simulink model "QuadCopter"  (R2024a)
settings: Solver=VariableStepAuto  StartTime=0.0  StopTime=Tsim  RelTol=1e-3
values from neighbouring files (symbols this model uses):
  l = size(Aa,2)    [RobustControl.m]
undefined symbols (not defined in the file or in its folder): b, d, g, Ixx, Iyy, Izz, Jr, m, x0
settings Model: Creator=giuco  LastModifiedBy=giuco

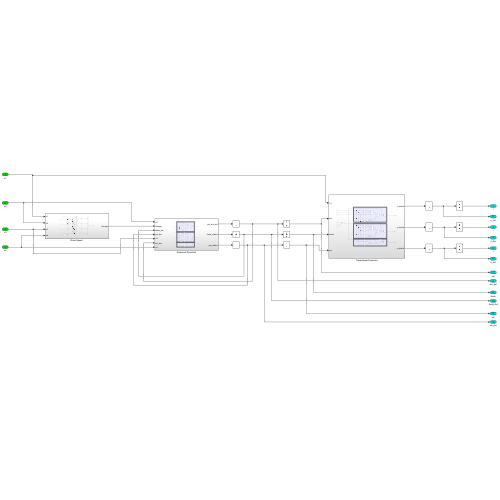
[thumbnail: Simulink's stored preview of the top-level diagram]
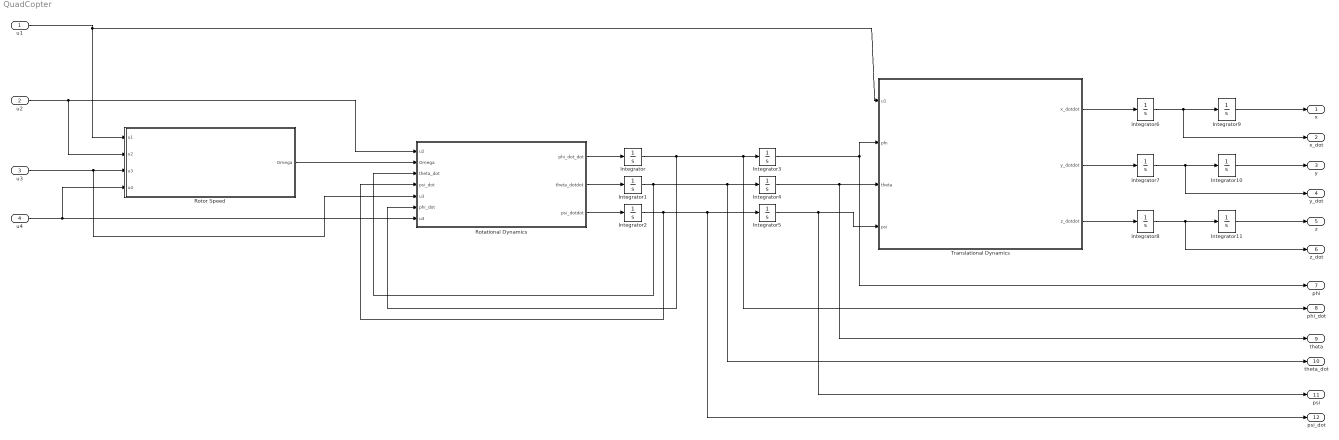
== system QuadCopter ==
  u1 : Inport
  u2 : Inport  Port=2
  u3 : Inport  Port=3
  u4 : Inport  Port=4
  Integrator : Integrator  InitialCondition=x0(2)
  Integrator1 : Integrator  InitialCondition=x0(4)
  Integrator10 : Integrator  InitialCondition=x0(9)
  Integrator11 : Integrator  InitialCondition=x0(11)
  Integrator2 : Integrator  InitialCondition=x0(6)
  Integrator3 : Integrator  InitialCondition=x0(1)
  Integrator4 : Integrator  InitialCondition=x0(3)
  Integrator5 : Integrator  InitialCondition=x0(5)
  Integrator6 : Integrator  InitialCondition=x0(8)
  Integrator7 : Integrator  InitialCondition=x0(10)
  Integrator8 : Integrator  InitialCondition=x0(12)
  Integrator9 : Integrator  InitialCondition=x0(7)
  Rotational Dynamics : Subsystem
  "Rotor Speed " : Subsystem
  Translational Dynamics : Subsystem
  x : Outport
  x_dot : Outport  Port=2
  y : Outport  Port=3
  y_dot : Outport  Port=4
  z : Outport  Port=5
  z_dot : Outport  Port=6
  phi : Outport  Port=7
  phi_dot : Outport  Port=8
  theta : Outport  Port=9
  theta_dot : Outport  Port=10
  psi : Outport  Port=11
  psi_dot : Outport  Port=12
  wires:
  u4/1 -> Rotational Dynamics/7(u4), "Rotor Speed "/4(u4)
  u2/1 -> Rotational Dynamics/1(u2), "Rotor Speed "/2(u2)
  Rotational Dynamics/1(phi_dot_dot) -> Integrator/1
  "Rotor Speed "/1(Omega) -> Rotational Dynamics/2(Omega)
  Integrator4/1 -> theta/1, Translational Dynamics/3(theta)
  Translational Dynamics/1(x_dotdot) -> Integrator6/1
  Rotational Dynamics/2(theta_dotdot) -> Integrator1/1
  Integrator5/1 -> psi/1, Translational Dynamics/4(psi)
  u1/1 -> "Rotor Speed "/1(u1), Translational Dynamics/1(u1)
  Integrator7/1 -> y_dot/1, Integrator10/1
  Integrator3/1 -> phi/1, Translational Dynamics/2(phi)
  Translational Dynamics/2(y_dotdot) -> Integrator7/1
  Integrator9/1 -> x/1
  Integrator1/1 -> theta_dot/1, Integrator4/1, Rotational Dynamics/3(theta_dot)
  Integrator10/1 -> y/1
  Integrator2/1 -> psi_dot/1, Integrator5/1, Rotational Dynamics/4(psi_dot)
  u3/1 -> "Rotor Speed "/3(u3), Rotational Dynamics/5(u3)
  Integrator6/1 -> x_dot/1, Integrator9/1
  Integrator/1 -> Rotational Dynamics/6(phi_dot), phi_dot/1, Integrator3/1
  Integrator8/1 -> z_dot/1, Integrator11/1
  Rotational Dynamics/3(psi_dotdot) -> Integrator2/1
  Translational Dynamics/3(z_dotdot) -> Integrator8/1
  Integrator11/1 -> z/1

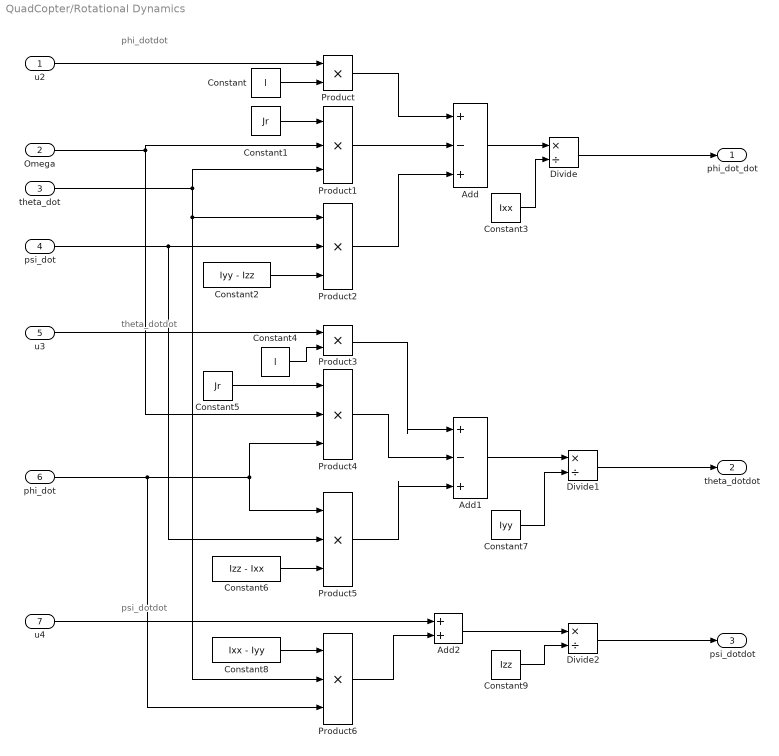
== system QuadCopter/Rotational Dynamics ==
  note: phi_dotdot
  note: theta_dotdot
  note: psi_dotdot
  u2 : Inport
  Omega : Inport  Port=2
  theta_dot : Inport  Port=3
  psi_dot : Inport  Port=4
  u3 : Inport  Port=5
  phi_dot : Inport  Port=6
  u4 : Inport  Port=7
  Add : Sum  Inputs=+-+
  Add1 : Sum  Inputs=+-+
  Add2 : Sum
  Constant : Constant  Value=l
  Constant1 : Constant  Value=Jr
  Constant2 : Constant  Value=Iyy - Izz
  Constant3 : Constant  Value=Ixx
  Constant4 : Constant  Value=l
  Constant5 : Constant  Value=Jr
  Constant6 : Constant  Value=Izz - Ixx
  Constant7 : Constant  Value=Iyy
  Constant8 : Constant  Value=Ixx - Iyy
  Constant9 : Constant  Value=Izz
  Divide : Product  Inputs=*/
  Divide1 : Product  Inputs=*/
  Divide2 : Product  Inputs=*/
  Product : Product
  Product{1..2,4..6} (5 alike) : Product  Inputs=3
  Product3 : Product
  phi_dot_dot : Outport
  theta_dotdot : Outport  Port=2
  psi_dotdot : Outport  Port=3
  wires:
  u2/1 -> Product/1
  Constant/1 -> Product/2
  Omega/1 -> Product1/2, Product4/2
  Constant1/1 -> Product1/1
  theta_dot/1 -> Product1/3, Product2/1, Product6/2
  psi_dot/1 -> Product5/2, Product2/2
  Constant2/1 -> Product2/3
  Product1/1 -> Add/2
  Product/1 -> Add/1
  Product2/1 -> Add/3
  Add/1 -> Divide/1
  Divide/1 -> phi_dot_dot/1
  Constant3/1 -> Divide/2
  u3/1 -> Product3/1
  Constant4/1 -> Product3/2
  Constant5/1 -> Product4/1
  phi_dot/1 -> Product4/3, Product5/1, Product6/3
  Constant6/1 -> Product5/3
  Product4/1 -> Add1/2
  Product3/1 -> Add1/1
  Product5/1 -> Add1/3
  Add1/1 -> Divide1/1
  Constant7/1 -> Divide1/2
  Divide1/1 -> theta_dotdot/1
  Constant8/1 -> Product6/1
  u4/1 -> Add2/1
  Product6/1 -> Add2/2
  Add2/1 -> Divide2/1
  Constant9/1 -> Divide2/2
  Divide2/1 -> psi_dotdot/1

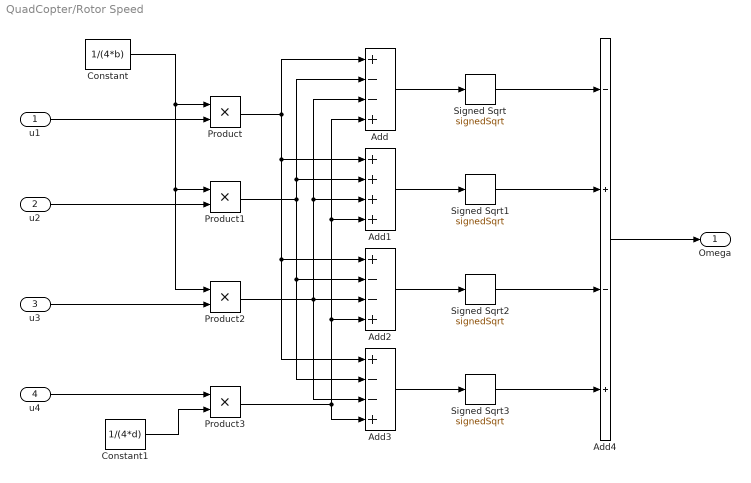
== system QuadCopter/Rotor Speed  ==
  u1 : Inport
  u2 : Inport  Port=2
  u3 : Inport  Port=3
  u4 : Inport  Port=4
  Add : Sum  Inputs=+--+
  Add1 : Sum  Inputs=++++
  Add2 : Sum  Inputs=+--+
  Add3 : Sum  Inputs=+--+
  Add4 : Sum  Inputs=-+-+
  Constant : Constant  Value=1/(4*b)
  Constant1 : Constant  Value=1/(4*d)
  Product{,1..3} (4 alike) : Product
  Signed Sqrt{,1..3} (4 alike) : Sqrt  Operator=signedSqrt
  Omega : Outport
  wires:
  u1/1 -> Product/2
  Constant/1 -> Product/1, Product1/1, Product2/1
  u2/1 -> Product1/2
  u3/1 -> Product2/2
  u4/1 -> Product3/1
  Constant1/1 -> Product3/2
  Product/1 -> Add3/1, Add2/1, Add1/1, Add/1
  Product1/1 -> Add2/2, Add3/2, Add1/2, Add/2
  Product2/1 -> Add2/3, Add1/3, Add/3, Add3/3
  Product3/1 -> Add3/4, Add2/4, Add/4, Add1/4
  Add/1 -> Signed Sqrt/1
  Add1/1 -> Signed Sqrt1/1
  Add2/1 -> Signed Sqrt2/1
  Add3/1 -> Signed Sqrt3/1
  Signed Sqrt/1 -> Add4/1
  Signed Sqrt1/1 -> Add4/2
  Signed Sqrt2/1 -> Add4/3
  Signed Sqrt3/1 -> Add4/4
  Add4/1 -> Omega/1

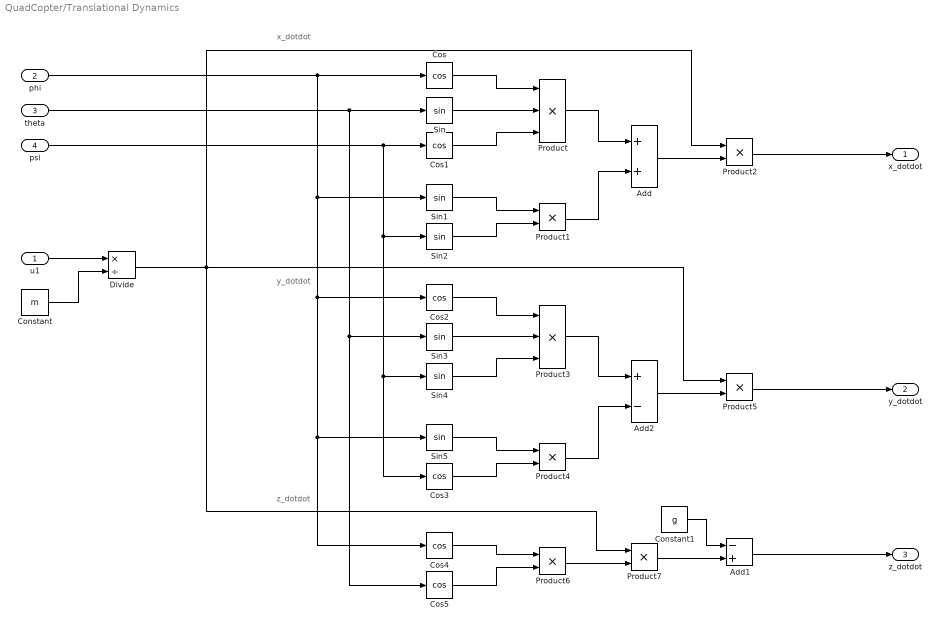
== system QuadCopter/Translational Dynamics ==
  note: x_dotdot
  note: y_dotdot
  note: z_dotdot
  u1 : Inport
  phi : Inport  Port=2
  theta : Inport  Port=3
  psi : Inport  Port=4
  Add : Sum
  Add1 : Sum  Inputs=-+
  Add2 : Sum  Inputs=+-
  Constant : Constant  Value=m
  Constant1 : Constant  Value=g
  Cos{,1..5} (6 alike) : Trigonometry  Operator=cos
  Divide : Product  Inputs=*/
  Product : Product  Inputs=3
  Product{1..2,4..7} (6 alike) : Product
  Product3 : Product  Inputs=3
  Sin{,1..5} (6 alike) : Trigonometry
  x_dotdot : Outport
  y_dotdot : Outport  Port=2
  z_dotdot : Outport  Port=3
  wires:
  u1/1 -> Divide/1
  Constant/1 -> Divide/2
  Divide/1 -> Product5/1, Product7/1, Product2/1
  phi/1 -> Cos/1, Sin1/1, Sin5/1, Cos4/1, Cos2/1
  theta/1 -> Sin/1, Sin3/1, Cos5/1
  psi/1 -> Cos1/1, Cos3/1, Sin4/1, Sin2/1
  Sin/1 -> Product/2
  Cos/1 -> Product/1
  Cos1/1 -> Product/3
  Sin1/1 -> Product1/1
  Sin2/1 -> Product1/2
  Product1/1 -> Add/2
  Product/1 -> Add/1
  Add/1 -> Product2/2
  Product2/1 -> x_dotdot/1
  Sin3/1 -> Product3/2
  Cos2/1 -> Product3/1
  Sin4/1 -> Product3/3
  Cos3/1 -> Product4/2
  Sin5/1 -> Product4/1
  Product4/1 -> Add2/2
  Product3/1 -> Add2/1
  Add2/1 -> Product5/2
  Product5/1 -> y_dotdot/1
  Cos4/1 -> Product6/1
  Cos5/1 -> Product6/2
  Product6/1 -> Product7/2
  Product7/1 -> Add1/2
  Constant1/1 -> Add1/1
  Add1/1 -> z_dotdot/1
